simulink model "ModeLogic"  (R2025b)
settings: configuration reference "mdlCheck_config_allPass" (kept outside this file)
settings Model: DataDictionary=ModeLogic_data.sldd  Creator=manthony  LastModifiedBy=patcanny
settings ConfigSetRef: SourceName=mdlCheck_config_allPass

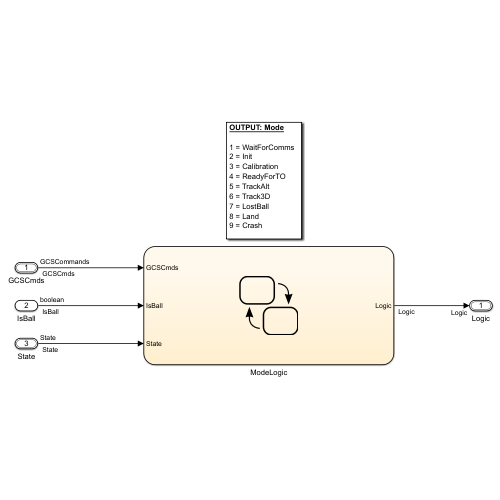
[thumbnail: Simulink's stored preview of the top-level diagram]
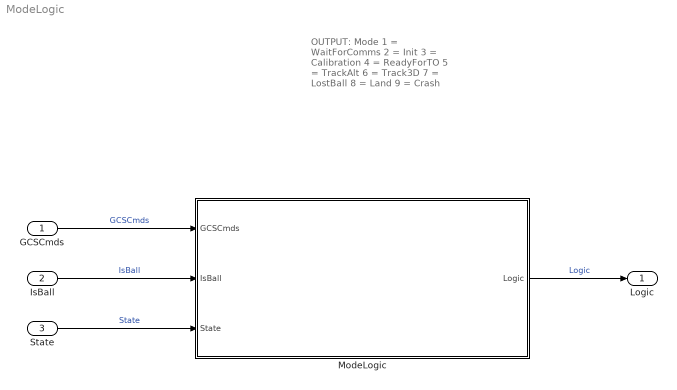
== system ModeLogic ==
  note: OUTPUT: Mode
      |
      | 1 = WaitForComms
      | 2 = Init
      | 3 = Calibration
      | 4 = ReadyForTO
      | 5 = TrackAlt
      | 6 = Track3D
      | 7 = LostBall
      | 8 = Land
      | 9 = Crash
  GCSCmds : Inport  OutDataTypeStr=Bus: GCSCommands  PortDimensions=1  SampleTime=0.1  Interpolate=off  BusOutputAsStruct=on
  IsBall : Inport  Port=2  OutDataTypeStr=boolean  PortDimensions=1  SampleTime=0.1  Interpolate=off
  State : Inport  Port=3  OutDataTypeStr=Bus: State  PortDimensions=1  SampleTime=0.1  Interpolate=off  BusOutputAsStruct=on
  ModeLogic : Stateflow chart  TreatAsAtomicUnit=on
      settings: RTWSystemCode=Inline
  Logic : Outport  OutDataTypeStr=Bus: Logic  PortDimensions=1  SampleTime=0.1  VectorParamsAs1DForOutWhenUnconnected=off  BusOutputAsStruct=on
  wires:
  GCSCmds/1 -> ModeLogic/1(GCSCmds)  "GCSCmds"
  State/1 -> ModeLogic/3(State)  "State"
  IsBall/1 -> ModeLogic/2(IsBall)  "IsBall"
  ModeLogic/1(Logic) -> Logic/1  "Logic"

== stateflow chart ModeLogic/ModeLogic ==
  settings: sampleTime=0.01  executeAtInitialization=1
  note: INPUT: GCS_MissionMode
      |
      | 0 = PowerUp/Standby
      | 1 = TrackBall
      | 2 = Land
  note: OUTPUT: Mode
      |
      | 1 = WaitForComms
      | 2 = Init
      | 3 = Calibration
      | 4 = ReadyForTO
      | 5 = TrackAlt
      | 6 = Track3D
      | 7 = LostBall
      | 8 = Land
      | 9 = Crash
  state WaitForComms
    en:
    Logic.Mode =  uint8(1);
  state Init
    en:
    Logic.Mode =  uint8(2);
  state Crash
    en:
    Logic.Mode = uint8(9);
  state Calibration
    en:
    Logic.Mode =  uint8(3);
    Logic.CalibrateSensors = true;
    du:
    Logic.CalibrateSensors = false;
  state ReadyForTO
    en:
    Logic.Mode =  uint8(4);
  state TrackAlt
    en:
    Logic.Mode =  uint8(5);
  state Track3D
    en:
    Logic.Mode =  uint8(6);
  state Land
    en:
    Logic.Mode = uint8(8);
  state LostBall
    en:
    Logic.Mode =  uint8(7);
  (default) -> WaitForComms
  (junction 95) -> WaitForComms
  Land -> (junction 95) [order 1] : [abs(State.Angles[0])*single(180)/single(3.1415) < single(5) && ...
      | abs(State.Angles[1])*single(180)/single(3.1415) < single(5) && ...
      | abs(State.V_BODY[2]) < single(0.1) ]
  Crash -> (junction 95)
  WaitForComms -> Init : [GCSCmds.WIFIconnected && GCSCmds.BTconnected]
  Init -> Calibration : [GCSCmds.CalibrateCmd]
  (junction 82) -> Crash : /*1.39626 rad ~= 80 deg */
      | [GCSCmds.EMERGENCY_OFF || ...
      | abs(State.Angles[0]) > single(1.39626) || ...
      | abs(State.Angles[1]) > single(1.39626)]
  ReadyForTO -> Calibration [order 2] : [GCSCmds.CalibrateCmd]
  TrackAlt -> (junction 82) [order 1]
  Land -> (junction 82) [order 2]
  LostBall -> (junction 82) [order 3]
  Track3D -> (junction 82) [order 2]
  Calibration -> ReadyForTO : [GCSCmds.GCS_MissionMode == uint8(1) && ...
      | State.CalibrationDone]
  ReadyForTO -> TrackAlt [order 1] : [IsBall]
  TrackAlt -> Track3D [order 2] : [State.Altitude >= single(0.1)]
  TrackAlt -> (junction 91) [order 3]
  (junction 101) -> TrackAlt [order 2]
  (junction 101) -> Track3D [order 1] : [State.Altitude >= single(0.1)]
  Track3D -> (junction 91) [order 1]
  LostBall -> (junction 101) [order 2] : [IsBall]
  (junction 91) -> Land [order 1] : [GCSCmds.GCS_MissionMode == uint8(2) || ...
      | State.BatteryVolts <= single(3)]
  (junction 91) -> LostBall [order 2] : [~IsBall]
  LostBall -> Land [order 1] : [count >= uint8(29)]
  LostBall -> LostBall [order 4] : {count = count+uint8(1);}
  data: Logic output Bus: Logic size=1; GCSCmds input Bus: GCSCommands; IsBall input boolean; State input Bus: State; count local uint8 size=1 =uint16(0)
